simulink model "stance2"  (R2014b)
settings: Solver=ode3  StartTime=0.0  StopTime=10.0  FixedStep=.001  MaxStep=ts_max  RelTol=1e-3  AbsTol=1e-4
values from neighbouring files (symbols this model uses):
  c = 0.05    [hopper.m]
  d = .04    (= 0.04)    [hopper.m]
  dp = .015    (= 0.015)    [hopper.m]
  eref = .04    (= 0.04)    [hopper.m]
  Fmax = 22000    [hopper.m]
  G = 1.07/Fmax    (= 4.86363636364e-05)    [hopper.m]
  K = 5    [hopper.m]
  lopt = .1    (= 0.1)    [hopper.m]
  lref = .5    (= 0.5)    [hopper.m]
  lrest = .4    (= 0.4)    [hopper.m]
  Ls = .5    (= 0.5)    [hopper.m]
  m = 80    [hopper.m]
  N = 1.5    [hopper.m]
  phiref = 110/180*pi    (= 1.91986217719)    [hopper.m]
  stances = yFspeed(end)    [hopper.m]
  stancey = yF(end)    [hopper.m]
  stm0 = .05    (= 0.05)    [hopper.m]
  Vmax = 12    [hopper.m]
  w = .4    (= 0.4)    [hopper.m]
libraries: simulink_extras x1
settings Model: Creator=hamidreza  LastModifiedBy=hamidreza

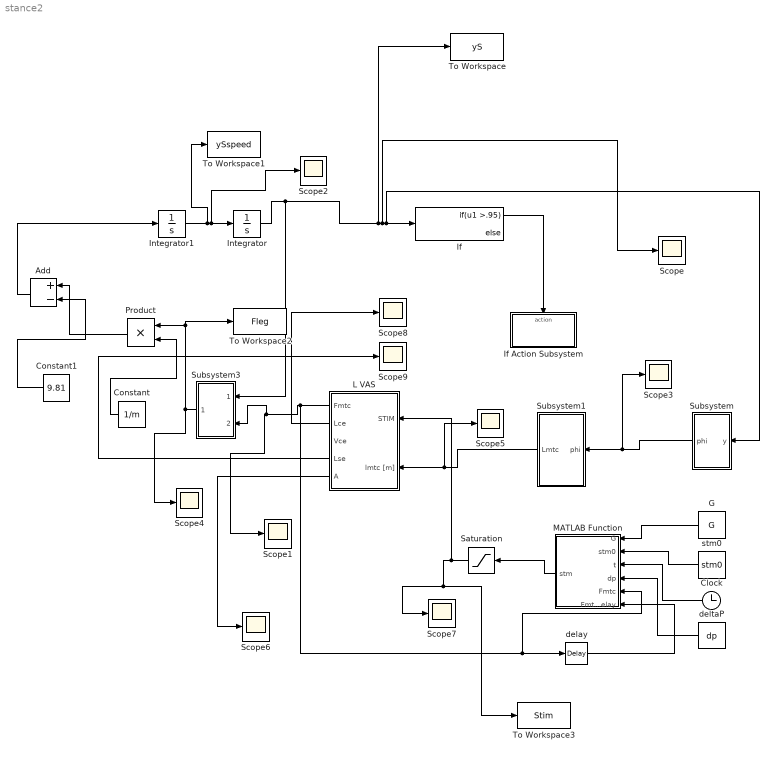
== system stance2 ==
  Add : Sum  Inputs=+-
  Clock : Clock
  Constant : Constant  Value=1/m
  Constant1 : Constant  Value=9.81
  G : Constant  Value=G
  If : If  IfExpression=u1 >.95
  If Action Subsystem : Subsystem  TreatAsAtomicUnit=on
  Integrator : Integrator  InitialCondition=stancey
  Integrator1 : Integrator  InitialCondition=stances
  L VAS : Subsystem
  MATLAB Function : MATLAB Function  TreatAsAtomicUnit=on
  Product : Product
  Saturation : Saturate  UpperLimit=1  LowerLimit=0
  Scope{,1..9} (10 alike) : Scope
      Scope settings: TimeRange=4.997999999999995  YMin=0  YMax=3.5
      Scope1 settings: TimeRange=1.285973939697051  YMin=0  YMax=2000
      Scope2 settings: TimeRange=4.997999999999995  YMin=0  YMax=3.5  SaveName=ScopeData2
      Scope3 settings: TimeRange=4.997999999999995  YMin=0  YMax=3.5  SaveName=ScopeData3
      Scope4 settings: TimeRange=1.285973939697051  YMin=0  YMax=2000  SaveName=ScopeData4
      Scope5 settings: TimeRange=4.997999999999995  YMin=0  YMax=3.5  SaveName=ScopeData5
      Scope6 settings: TimeRange=4.997999999999995  YMin=0  YMax=3.5  SaveName=ScopeData6
      Scope7 settings: TimeRange=4.997999999999995  YMin=0  YMax=3.5  SaveName=ScopeData7
      Scope8 settings: TimeRange=4.997999999999995  YMin=0  YMax=3.5  SaveName=ScopeData8
      Scope9 settings: TimeRange=4.997999999999995  YMin=0  YMax=3.5  SaveName=ScopeData9
  Subsystem : Subsystem
  Subsystem1 : Subsystem
  Subsystem3 : Subsystem
  To Workspace : ToWorkspace  VariableName=yS  SaveFormat=Structure With Time  SampleTime=-1
  To Workspace1 : ToWorkspace  VariableName=ySspeed  SaveFormat=Structure With Time  SampleTime=-1
  To Workspace2 : ToWorkspace  VariableName=Fleg  SaveFormat=Structure With Time  SampleTime=-1
  To Workspace3 : ToWorkspace  VariableName=Stim  SaveFormat=Structure With Time  SampleTime=-1
  "delay " : TransportDelay  DelayTime=.015
  deltaP : Constant  Value=dp
  stm0 : Constant  Value=stm0
  wires:
  Integrator/1 -> Subsystem3/1(lLeg), If/1, Subsystem/1(y), Scope/1, To Workspace/1
  Integrator1/1 -> To Workspace1/1, Scope2/1, Integrator/1
  If/1 -> If Action Subsystem/Action
  Constant/1 -> Product/2
  Subsystem/1("phi ") -> Scope3/1, Subsystem1/1(phi)
  Subsystem1/1(Lmtc) -> Scope5/1, L VAS/2(lmtc [m])
  G/1 -> MATLAB Function/1(G)
  stm0/1 -> MATLAB Function/2(stm0)
  Clock/1 -> MATLAB Function/3(t)
  deltaP/1 -> MATLAB Function/4(dp)
  Saturation/1 -> To Workspace3/1, Scope7/1, L VAS/1(STIM)
  L VAS/1(Fmtc) -> MATLAB Function/5(Fmtc), "delay "/1, Subsystem3/2(Fmtc), Scope1/1
  Product/1 -> Add/1
  Constant1/1 -> Add/2
  Add/1 -> Integrator1/1
  L VAS/5(A) -> Scope6/1
  Subsystem3/1(Fleg) -> To Workspace2/1, Product/1, Scope4/1
  L VAS/2(Lce) -> Scope8/1
  L VAS/4(Lse) -> Scope9/1
  MATLAB Function/1(stm) -> Saturation/1
  "delay "/1 -> MATLAB Function/6(Fmtcdelay)

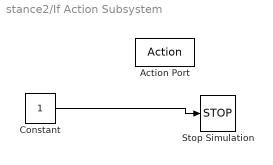
== system stance2/If Action Subsystem ==
  Action Port : ActionPort  ActionType=then
  Constant : Constant
  Stop Simulation : Stop
  wires:
  Constant/1 -> Stop Simulation/1

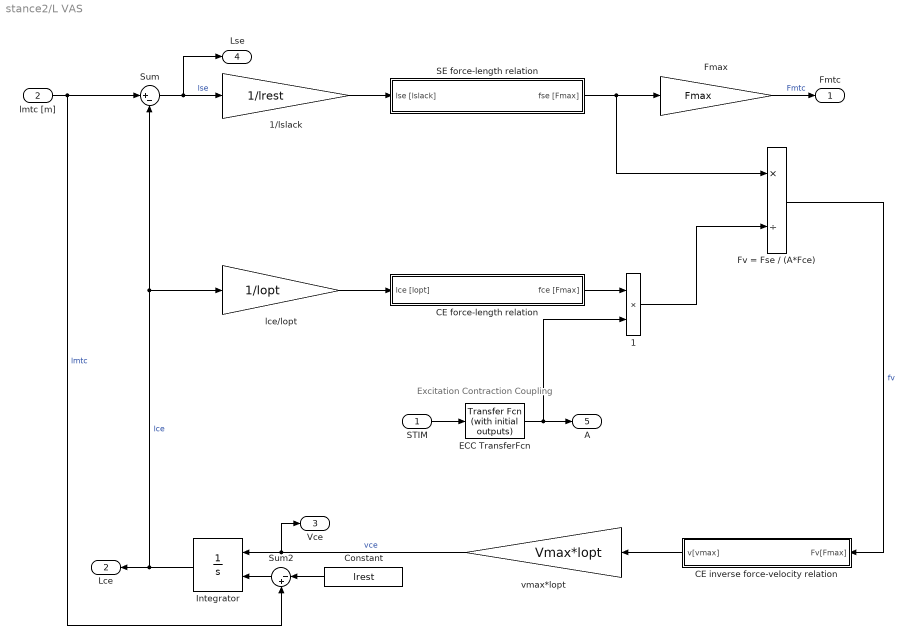
== system stance2/L VAS ==
  note: Excitation Contraction Coupling
  STIM : Inport
  lmtc [m] : Inport  Port=2
  1 : Product  Inputs=**  SaturateOnIntegerOverflow=on  InputSameDT=on  OutDataTypeStr=Inherit: Same as first input
  1/lslack : Gain  Gain=1/lrest  SaturateOnIntegerOverflow=on  OutDataTypeStr=Inherit: Same as input  ParamDataTypeStr=Inherit: Same as input
  CE force-length relation : Subsystem
  CE inverse force-velocity relation : Subsystem
  Constant : Constant  Value=lrest
  ECC TransferFcn : simulink_extras/Additional Linear/Transfer Fcn (with initial outputs)  N=[1]  D="[.01  1]"  Y0=preA  U0=0
      settings: AttributesFormatString=pre-activation: %<Y0>
  Fmax : Gain  Gain=Fmax  SaturateOnIntegerOverflow=on  OutDataTypeStr=Inherit: Same as input  ParamDataTypeStr=Inherit: Same as input
  Fv = Fse / (A*Fce) : Product  Inputs=*/  SaturateOnIntegerOverflow=on  InputSameDT=on  OutDataTypeStr=Inherit: Same as first input
  Integrator : Integrator  InitialConditionSource=external  LowerSaturationLimit=0.05
  SE force-length relation : Subsystem
  Sum : Sum  Inputs=|+-  SaturateOnIntegerOverflow=on  InputSameDT=on  OutDataTypeStr=Inherit: Same as first input
  Sum2 : Sum  Inputs=|-+  SaturateOnIntegerOverflow=on  InputSameDT=on  OutDataTypeStr=Inherit: Same as first input
  lce/lopt : Gain  Gain=1/lopt  SaturateOnIntegerOverflow=on  OutDataTypeStr=Inherit: Same as input  ParamDataTypeStr=Inherit: Same as input
  vmax*lopt : Gain  Gain=Vmax*lopt  SaturateOnIntegerOverflow=on  OutDataTypeStr=Inherit: Same as input  ParamDataTypeStr=Inherit: Same as input
  Fmtc : Outport  InitialOutput=0
  Lce : Outport  Port=2  InitialOutput=0
  Vce : Outport  Port=3  InitialOutput=0
  Lse : Outport  Port=4  InitialOutput=0
  A : Outport  Port=5  InitialOutput=0
  wires:
  Integrator/1 -> Sum/2, lce/lopt/1, Lce/1  "lce"
  Sum/1 -> 1/lslack/1, Lse/1  "lse"
  lce/lopt/1 -> CE force-length relation/1(lce [lopt])
  Fv = Fse / (A*Fce)/1 -> CE inverse force-velocity relation/1(Fv[Fmax])  "fv"
  vmax*lopt/1 -> Integrator/1, Vce/1  "vce"
  lmtc [m]/1 -> Sum2/2, Sum/1  "lmtc"
  Fmax/1 -> Fmtc/1  "Fmtc"
  1/lslack/1 -> SE force-length relation/1(lse [lslack])
  Sum2/1 -> Integrator/2
  Constant/1 -> Sum2/1
  CE force-length relation/1(fce [Fmax]) -> 1/1
  SE force-length relation/1(fse [Fmax]) -> Fmax/1, Fv = Fse / (A*Fce)/1
  1/1 -> Fv = Fse / (A*Fce)/2
  CE inverse force-velocity relation/1(v[vmax]) -> vmax*lopt/1
  STIM/1 -> ECC TransferFcn/1
  ECC TransferFcn/1 -> 1/2, A/1

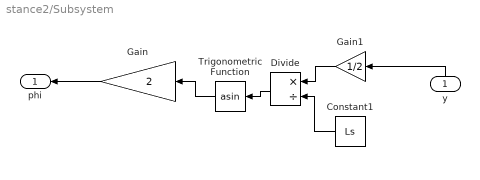
== system stance2/Subsystem ==
  y : Inport
  Constant1 : Constant  Value=Ls
  Divide : Product  Inputs=*/
  Gain : Gain  Gain=2
  Gain1 : Gain  Gain=1/2
  Trigonometric Function : Trigonometry  Operator=asin
  "phi " : Outport
  wires:
  Trigonometric Function/1 -> Gain/1
  Divide/1 -> Trigonometric Function/1
  y/1 -> Gain1/1
  Constant1/1 -> Divide/2
  Gain1/1 -> Divide/1
  Gain/1 -> "phi "/1

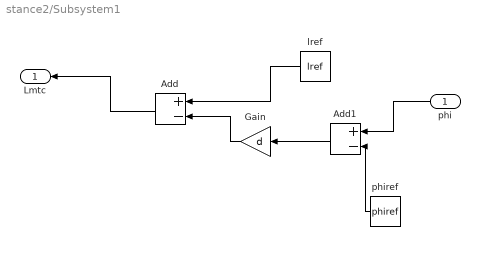
== system stance2/Subsystem1 ==
  phi : Inport
  Add : Sum  Inputs=+-
  Add1 : Sum  Inputs=+-
  Gain : Gain  Gain=d
  lref : Constant  Value=lref
  phiref : Constant  Value=phiref
  Lmtc : Outport
  wires:
  phiref/1 -> Add1/2
  phi/1 -> Add1/1
  lref/1 -> Add/1
  Gain/1 -> Add/2
  Add1/1 -> Gain/1
  Add/1 -> Lmtc/1

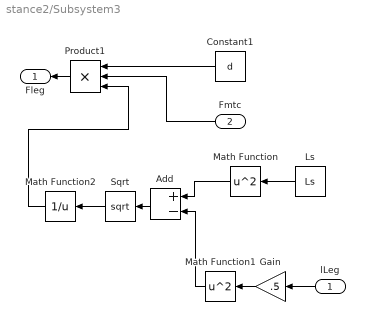
== system stance2/Subsystem3 ==
  lLeg : Inport
  Fmtc : Inport  Port=2
  Add : Sum  Inputs=+-
  Constant1 : Constant  Value=d
  Gain : Gain  Gain=.5
  Ls : Constant  Value=Ls
  Math Function : Math  Operator=square  SaturateOnIntegerOverflow=on
  Math Function1 : Math  Operator=square  SaturateOnIntegerOverflow=on
  Math Function2 : Math  Operator=reciprocal  SaturateOnIntegerOverflow=on
  Product1 : Product  Inputs=3
  Sqrt : Sqrt  SaturateOnIntegerOverflow=on
  Fleg : Outport
  wires:
  Product1/1 -> Fleg/1
  Math Function1/1 -> Add/2
  Ls/1 -> Math Function/1
  lLeg/1 -> Gain/1
  Fmtc/1 -> Product1/2
  Constant1/1 -> Product1/1
  Sqrt/1 -> Math Function2/1
  Add/1 -> Sqrt/1
  Math Function/1 -> Add/1
  Math Function2/1 -> Product1/3
  Gain/1 -> Math Function1/1

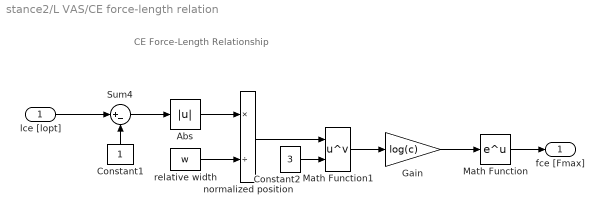
== system stance2/L VAS/CE force-length relation ==
  note: CE Force-Length Relationship
  lce [lopt] : Inport
  Abs : Abs
  Constant1 : Constant
  Constant2 : Constant  Value=3
  Gain : Gain  Gain=log(c)
  Math Function : Math  SaturateOnIntegerOverflow=on
  Math Function1 : Math  Operator=pow  SaturateOnIntegerOverflow=on
  Sum4 : Sum  Inputs=|+-  SaturateOnIntegerOverflow=on  InputSameDT=on  OutDataTypeStr=Inherit: Same as first input
  normalized position : Product  Inputs=*/
  relative width : Constant  Value=w
  fce [Fmax] : Outport
  wires:
  lce [lopt]/1 -> Sum4/1
  relative width/1 -> normalized position/2
  Constant1/1 -> Sum4/2
  Sum4/1 -> Abs/1
  Abs/1 -> normalized position/1
  normalized position/1 -> Math Function1/1
  Constant2/1 -> Math Function1/2
  Math Function1/1 -> Gain/1
  Gain/1 -> Math Function/1
  Math Function/1 -> fce [Fmax]/1

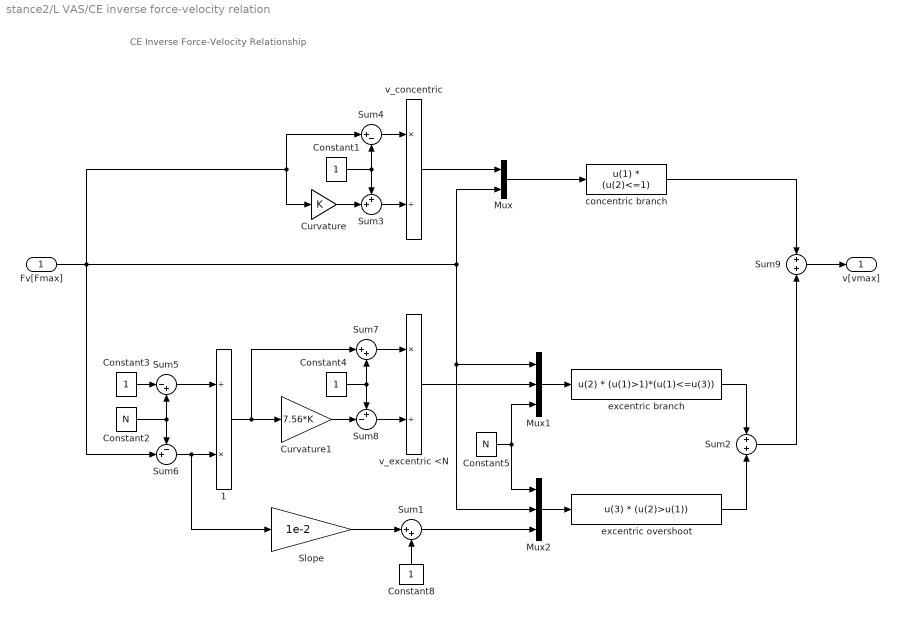
== system stance2/L VAS/CE inverse force-velocity relation ==
  note: CE Inverse Force-Velocity Relationship
  Fv[Fmax] : Inport
  1 : Product  Inputs=/*
  Constant{1,3..4,8} (4 alike) : Constant
  Constant2 : Constant  Value=N
  Constant5 : Constant  Value=N
  Curvature : Gain  Gain=K  SaturateOnIntegerOverflow=on  OutDataTypeStr=Inherit: Same as input  ParamDataTypeStr=Inherit: Same as input
  Curvature1 : Gain  Gain=7.56*K  SaturateOnIntegerOverflow=on  OutDataTypeStr=Inherit: Same as input  ParamDataTypeStr=Inherit: Same as input
  Mux : Mux  Inputs=2
  Mux1 : Mux  Inputs=3
  Mux2 : Mux  Inputs=3
  Slope : Gain  Gain=1e-2  SaturateOnIntegerOverflow=on  OutDataTypeStr=Inherit: Same as input  ParamDataTypeStr=Inherit: Same as input
  Sum1 : Sum  Inputs=|++  SaturateOnIntegerOverflow=on  InputSameDT=on  OutDataTypeStr=Inherit: Same as first input
  Sum2 : Sum  SaturateOnIntegerOverflow=on  InputSameDT=on  OutDataTypeStr=Inherit: Same as first input
  Sum3 : Sum  Inputs=++|  SaturateOnIntegerOverflow=on  InputSameDT=on  OutDataTypeStr=Inherit: Same as first input
  Sum4 : Sum  Inputs=|+-  SaturateOnIntegerOverflow=on  InputSameDT=on  OutDataTypeStr=Inherit: Same as first input
  Sum5 : Sum  Inputs=|-+  SaturateOnIntegerOverflow=on  InputSameDT=on  OutDataTypeStr=Inherit: Same as first input
  Sum6 : Sum  Inputs=-+|  SaturateOnIntegerOverflow=on  InputSameDT=on  OutDataTypeStr=Inherit: Same as first input
  Sum7 : Sum  Inputs=|++  SaturateOnIntegerOverflow=on  InputSameDT=on  OutDataTypeStr=Inherit: Same as first input
  Sum8 : Sum  Inputs=+-|  SaturateOnIntegerOverflow=on  InputSameDT=on  OutDataTypeStr=Inherit: Same as first input
  Sum9 : Sum  SaturateOnIntegerOverflow=on  InputSameDT=on  OutDataTypeStr=Inherit: Same as first input
  concentric branch : Fcn  Expr=u(1) * (u(2)<=1)
  excentric branch : Fcn  Expr=u(2) * (u(1)>1)*(u(1)<=u(3))
  excentric overshoot : Fcn  Expr=u(3) * (u(2)>u(1))
  v_concentric : Product  Inputs=*/
  v_excentric <N : Product  Inputs=*/
  v[vmax] : Outport
  wires:
  Curvature/1 -> Sum3/2
  Constant1/1 -> Sum4/2, Sum3/1
  Sum4/1 -> v_concentric/1
  Sum3/1 -> v_concentric/2
  1/1 -> Sum7/1, Curvature1/1
  Constant4/1 -> Sum7/2, Sum8/1
  Curvature1/1 -> Sum8/2
  Sum8/1 -> v_excentric <N/2
  Sum7/1 -> v_excentric <N/1
  v_concentric/1 -> Mux/1
  Fv[Fmax]/1 -> Sum4/1, Curvature/1, Sum6/2, Mux/2, Mux1/1, Mux2/2
  Sum9/1 -> v[vmax]/1
  Sum2/1 -> Sum9/2
  excentric overshoot/1 -> Sum2/2
  Slope/1 -> Sum1/1
  Constant8/1 -> Sum1/2
  Sum6/1 -> 1/2, Slope/1
  Constant2/1 -> Sum6/1, Sum5/2
  Sum5/1 -> 1/1
  Constant3/1 -> Sum5/1
  Mux/1 -> concentric branch/1
  Mux1/1 -> excentric branch/1
  v_excentric <N/1 -> Mux1/2
  Mux2/1 -> excentric overshoot/1
  concentric branch/1 -> Sum9/1
  excentric branch/1 -> Sum2/1
  Constant5/1 -> Mux1/3, Mux2/1
  Sum1/1 -> Mux2/3

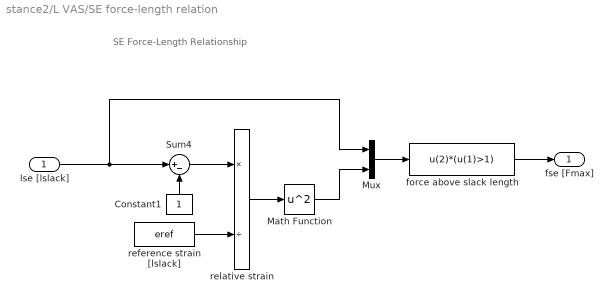
== system stance2/L VAS/SE force-length relation ==
  note: SE Force-Length Relationship
  lse [lslack] : Inport
  Constant1 : Constant
  Math Function : Math  Operator=square  SaturateOnIntegerOverflow=on
  Mux : Mux  Inputs=2
  Sum4 : Sum  Inputs=|+-  SaturateOnIntegerOverflow=on  InputSameDT=on  OutDataTypeStr=Inherit: Same as first input
  force above slack length : Fcn  Expr=u(2)*(u(1)>1)
  reference strain [lslack] : Constant  Value=eref
  relative strain : Product  Inputs=*/
  fse [Fmax] : Outport
  wires:
  Mux/1 -> force above slack length/1
  force above slack length/1 -> fse [Fmax]/1
  Math Function/1 -> Mux/2
  lse [lslack]/1 -> Mux/1, Sum4/1
  relative strain/1 -> Math Function/1
  reference strain [lslack]/1 -> relative strain/2
  Sum4/1 -> relative strain/1
  Constant1/1 -> Sum4/2

== matlab function stance2/MATLAB Function ==
  data: G input; stm output; stm0 input; t input; dp input; Fmtc input; Fmtcdelay input
function  stm= fcn(G,stm0,t,dp,Fmtc,Fmtcdelay)

% if t<dp
%     stm=stm0;
%     
% else
    
    stm=stm0+Fmtcdelay*G;
end
